simulink model "TestAttitudeControl"  (R2016b)
settings: Solver=VariableStepAuto  StartTime=0.0  StopTime=10  RelTol=1e-3
undefined symbols (not defined in the file): armed, ctrl_state, Initial, v_att_sp, v_control_mode
libraries: QuaternionLibrary x6, simulink_extras x2, simulink x1
(part 1 of 2)
settings Model: Creator=jban039  LastModifiedBy=jban039

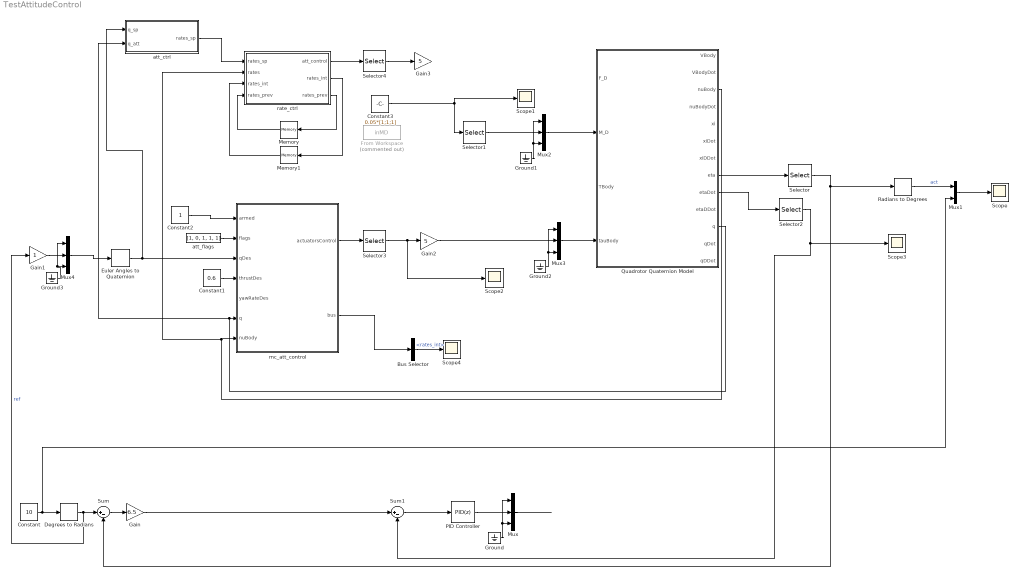
== system TestAttitudeControl ==
  Bus Selector : BusSelector  OutputSignals=rates_int
  Constant : Constant  Value=10
  Constant1 : Constant  Value=0.6
  Constant2 : Constant
  Constant3 : Constant  Value=0.05*[1;1;1]
  Degrees to Radians : simulink_extras/Transformations/Degrees to Radians
  Euler Angles to Quaternion : QuaternionLibrary/Euler Angles to Quaternion
  From Workspace : FromWorkspace  Commented=on  VariableName=inMD  SampleTime=0
  Gain : Gain  Gain=6.5
  Gain1 : Gain
  Gain2 : Gain  Gain=5
  Gain3 : Gain  Gain=5
  Ground{,1..3} (4 alike) : Ground
  Memory : Memory  X0=[0;0;0]
  Memory1 : Memory  X0=[0;0;0]
  Mux{,2..4} (4 alike) : Mux  Inputs=3
  Mux1 : Mux  Inputs=2
  PID Controller : simulink/Continuous/PID Controller  Controller=PID  TimeDomain=Discrete-time  SampleTime=0.004  IntegratorMethod=Forward Euler  FilterMethod=Forward Euler  Form=Parallel  UseFilter=off  ControllerParametersSource=internal  P=0.15  I=0.05  D=0.003  N=1000  InitialConditionSource=internal  InitialConditionForIntegrator=0  InitialConditionForFilter=0  ExternalReset=none  LimitOutput=off  UpperSaturationLimit=inf  LowerSaturationLimit=-inf  LinearizeAsGain=on  AntiWindupMode=none  Kb=1  TrackingMode=off  Kt=1  PParamMin=[]  PParamMax=[]  IParamMin=[]  IParamMax=[]  DParamMin=[]  DParamMax=[]  NParamMin=[]  NParamMax=[]  KbParamMin=[]  KbParamMax=[]  KtParamMin=[]  KtParamMax=[]  POutMin=[]  POutMax=[]  IOutMin=[]  IOutMax=[]  DOutMin=[]  DOutMax=[]  NOutMin=[]  NOutMax=[]  KbOutMin=[]  KbOutMax=[]  KtOutMin=[]  KtOutMax=[]  IntegratorOutMin=[]  IntegratorOutMax=[]  FilterOutMin=[]  FilterOutMax=[]  SumOutMin=[]  SumOutMax=[]  SumI1OutMin=[]  SumI1OutMax=[]  SumI2OutMin=[]  SumI2OutMax=[]  SumI3OutMin=[]  SumI3OutMax=[]  SumDOutMin=[]  SumDOutMax=[]  SaturationOutMin=[]  SaturationOutMax=[]  IntegratorContinuousStateAttributes=''  IntegratorStateMustResolveToSignalObject=off  IntegratorRTWStateStorageClass=Auto  FilterContinuousStateAttributes=''  FilterStateMustResolveToSignalObject=off  FilterRTWStateStorageClass=Auto  DifferentiatorICPrevScaledInput=0  DifferentiatorOutMin=[]  DifferentiatorOutMax=[]
  Quadrotor Quaternion Model : Subsystem
  Radians to Degrees : simulink_extras/Transformations/Radians to Degrees
  Scope{,1..4} (5 alike) : Scope
  Selector{,1..2,4} (4 alike) : Selector  InputPortWidth=3  IndexOptions=Index vector (dialog)  Indices=2  OutputSizes=1
  Selector3 : Selector  InputPortWidth=8  IndexOptions=Index vector (dialog)  Indices=2  OutputSizes=1
  Sum : Sum  Inputs=|+-
  Sum1 : Sum  Inputs=|+-
  att_ctrl : MATLAB Function  TreatAsAtomicUnit=on
  att_flags : Constant  Value=[1, 0, 1, 1, 1]
  mc_att_control : Subsystem  AncestorBlock=Px4Library/mc_att_control  mask(PX4 Attitude Controller: mc_att_control){MC_SAMPLING_PERIOD=0.004, MC_ROLL_TC=0.2, MC_PITCH_TC=0.2, MC_ROLL_P=6.5, MC_ROLLRATE_P=0.15, MC_ROLLRATE_I=0.05, MC_ROLLRATE_D=0.003, MC_ROLLRATE_FF=0, MC_PITCH_P=6.5, MC_PITCHRATE_P=0.15, MC_PITCHRATE_I=0.05, MC_PITCHRATE_D=0.003, MC_PITCHRATE_FF=0, MC_YAW_P=2.8, MC_YAWRATE_P=0.2, MC_YAWRATE_I=0.1, MC_YAWRATE_D=0, MC_YAWRATE_FF=0, MC_YAW_FF=0.5, MC_ROLLRATE_MAX=220, MC_PITCHRATE_MAX=220, MC_YAWRATE_MAX=200, MC_YAWRAUTO_MAX=45, MC_ACRO_R_MAX=360, MC_ACRO_P_MAX=360, MC_ACRO_Y_MAX=360, MC_RATT_TH=1, MC_TPA_BREAK=1, MC_TPA_SLOPE=1, VT_OPT_RECOV_EN=0, VT_WV_YAWR_SCL=0.15, MC_RR_INT_LIM=10.0, MC_PR_INT_LIM=10.0, MC_TPA_BREAK_P=1.0, MC_TPA_BREAK_I=1.0, MC_TPA_BREAK_D=1.0, MC_TPA_RATE_P=0.0, MC_TPA_RATE_I=0.0, MC_TPA_RATE_D=0.0, VT_TYPE=0, MC_BAT_SCALE_EN=0, MC_YR_INT_LIM=10.0}
      mask prompts: VT_TYPE "VT_TYPE (0 = Tailsitter, 1 = Tiltrotor, 2 = Standard)"
      mask help: Stabilization controller from the PX4 flight stack.
  rate_ctrl : MATLAB Function  TreatAsAtomicUnit=on  SystemSampleTime=0.002
  wires:
  Mux/1 -> ?
  Constant3/1 -> Selector1/1, Scope1/1
  Constant/1 -> Mux1/2, Degrees to Radians/1
  Sum/1 -> Gain/1
  Ground/1 -> Mux/1, Mux/3
  PID Controller/1 -> Mux/2
  Quadrotor Quaternion Model/8(eta) -> Selector/1
  Selector/1 -> Radians to Degrees/1, Sum/2
  Degrees to Radians/1 -> Gain1/1, Sum/1  "ref"
  Radians to Degrees/1 -> Mux1/1  "act"
  Mux1/1 -> Scope/1
  Ground1/1 -> Mux2/3, Mux2/1
  Selector1/1 -> Mux2/2
  Mux2/1 -> Quadrotor Quaternion Model/2(M_D)
  Quadrotor Quaternion Model/9(etaDot) -> Selector2/1
  Gain/1 -> Sum1/1
  Sum1/1 -> PID Controller/1
  mc_att_control/1(actuatorsControl) -> Selector3/1
  Euler Angles to Quaternion/1 -> att_ctrl/1(q_sp), mc_att_control/3(qDes)
  Constant1/1 -> mc_att_control/4(thrustDes)
  Quadrotor Quaternion Model/11(q) -> att_ctrl/2(q_att), mc_att_control/6(q)
  Quadrotor Quaternion Model/3(nuBody) -> rate_ctrl/2(rates), mc_att_control/7(nuBody)
  Constant2/1 -> mc_att_control/1(armed)
  att_flags/1 -> mc_att_control/2(flags)
  Mux3/1 -> Quadrotor Quaternion Model/4(tauBody)
  Ground2/1 -> Mux3/3, Mux3/1
  Selector3/1 -> Scope2/1, Gain2/1
  Mux4/1 -> Euler Angles to Quaternion/1
  Ground3/1 -> Mux4/1, Mux4/3
  Gain1/1 -> Mux4/2
  Gain2/1 -> Mux3/2
  Selector2/1 -> Scope3/1, Sum1/2
  att_ctrl/1(rates_sp) -> rate_ctrl/1(rates_sp)
  rate_ctrl/3(rates_prev) -> Memory/1
  Memory/1 -> rate_ctrl/4("rates_prev ")
  rate_ctrl/2(rates_int) -> Memory1/1
  Memory1/1 -> rate_ctrl/3("rates_int ")
  rate_ctrl/1(att_control) -> Selector4/1
  Selector4/1 -> Gain3/1
  mc_att_control/2(bus) -> Bus Selector/1
  Bus Selector/1 -> Scope4/1  "<rates_int>"

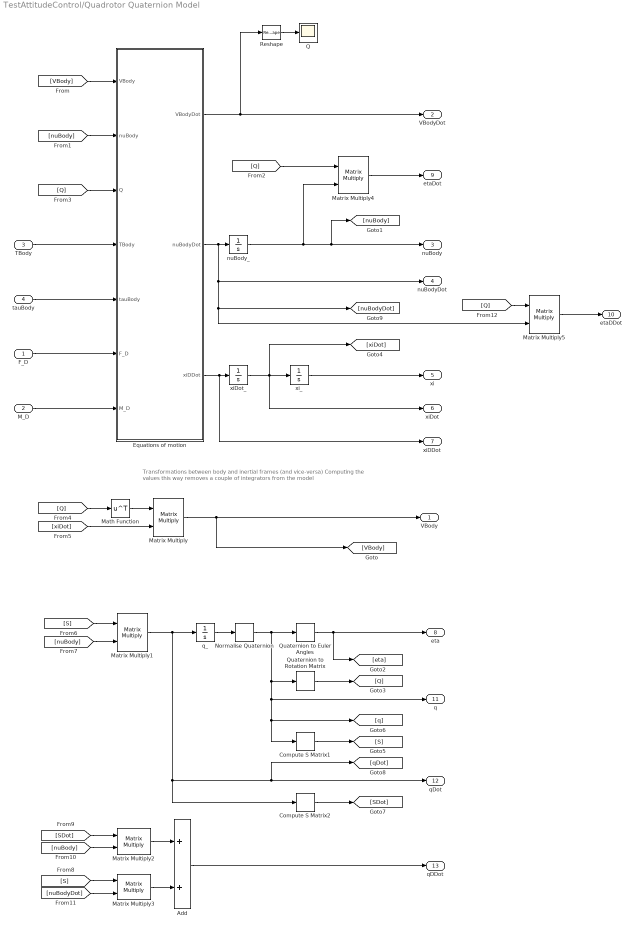
== system TestAttitudeControl/Quadrotor Quaternion Model ==
  note: Transformations between body and inertial frames (and vice-versa)
      | Computing the values this way removes a couple of integrators from the model
  F_D : Inport  Unit=N
  M_D : Inport  Port=2  Unit=N*m
  TBody : Inport  Port=3  Unit=N
  tauBody : Inport  Port=4  Unit=N*m
  Add : Sum
  Compute S Matrix1 : QuaternionLibrary/Compute S Matrix
  Compute S Matrix2 : QuaternionLibrary/Compute S Matrix
  Equations of motion : MATLAB Function  TreatAsAtomicUnit=on
  Math Function : Math  Operator=transpose  SaturateOnIntegerOverflow=on
  Matrix Multiply{,1..5} (6 alike) : Product  Multiplication=Matrix(*)
  Normalise Quaternion : QuaternionLibrary/Normalise Quaternion
  Q : Scope
  Quaternion to Euler Angles : QuaternionLibrary/Quaternion to Euler Angles
  Quaternion to Rotation Matrix : QuaternionLibrary/Quaternion to Rotation Matrix
  Reshape : Reshape  OutputDimensionality=Column vector (2-D)
  nuBody_ : Integrator  InitialCondition=Initial.NU_BODY
  q_ : Integrator  InitialCondition=Initial.Q
  xiDot_ : Integrator  InitialCondition=Initial.XI_DOT
  xi_ : Integrator  InitialCondition=Initial.XI
  VBody : Outport  Unit=m/s
  VBodyDot : Outport  Port=2  Unit=m/s^2
  nuBody : Outport  Port=3  Unit=rad/s
  nuBodyDot : Outport  Port=4  Unit=rad/s^2
  xi : Outport  Port=5  Unit=m
  xiDot : Outport  Port=6  Unit=m/s
  xiDDot : Outport  Port=7  Unit=m/s^2
  eta : Outport  Port=8  Unit=rad
  etaDot : Outport  Port=9  Unit=rad/s
  etaDDot : Outport  Port=10  Unit=rad/s^2
  q : Outport  Port=11
  qDot : Outport  Port=12
  qDDot : Outport  Port=13
  wires:
  Equations of motion/1(VBodyDot) -> Reshape/1, VBodyDot/1
  xi_/1 -> xi/1
  [nuBody] -> Equations of motion/2(nuBody)
  [VBody] -> Equations of motion/1(VBody)
  tauBody/1 -> Equations of motion/5(tauBody)
  TBody/1 -> Equations of motion/4(TBody)
  Equations of motion/3(xiDDot) -> xiDot_/1, xiDDot/1
  F_D/1 -> Equations of motion/6(F_D)
  Matrix Multiply/1 -> VBody/1, [VBody]
  M_D/1 -> Equations of motion/7(M_D)
  nuBody_/1 -> Matrix Multiply4/2, [nuBody], nuBody/1
  Equations of motion/2(nuBodyDot) -> nuBody_/1, nuBodyDot/1, Matrix Multiply5/2, [nuBodyDot]
  q_/1 -> Normalise Quaternion/1
  Quaternion to Euler Angles/1 -> eta/1, [eta]
  Matrix Multiply4/1 -> etaDot/1
  Quaternion to Rotation Matrix/1 -> [Q]
  [Q] -> Equations of motion/3(Q)
  [Q] -> Math Function/1
  [xiDot] -> Matrix Multiply/2
  Math Function/1 -> Matrix Multiply/1
  [S] -> Matrix Multiply1/1
  [nuBody] -> Matrix Multiply1/2
  Compute S Matrix2/1 -> [SDot]
  [S] -> Matrix Multiply3/1
  Matrix Multiply1/1 -> qDot/1, [qDot], Compute S Matrix2/1, q_/1
  [SDot] -> Matrix Multiply2/1
  [nuBody] -> Matrix Multiply2/2
  [nuBodyDot] -> Matrix Multiply3/2
  Matrix Multiply2/1 -> Add/1
  Matrix Multiply3/1 -> Add/2
  Normalise Quaternion/1 -> Quaternion to Euler Angles/1, q/1, Compute S Matrix1/1, [q], Quaternion to Rotation Matrix/1
  Compute S Matrix1/1 -> [S]
  [Q] -> Matrix Multiply4/1
  Add/1 -> qDDot/1
  [Q] -> Matrix Multiply5/1
  Matrix Multiply5/1 -> etaDDot/1
  Reshape/1 -> Q/1
  xiDot_/1 -> xi_/1, [xiDot], xiDot/1

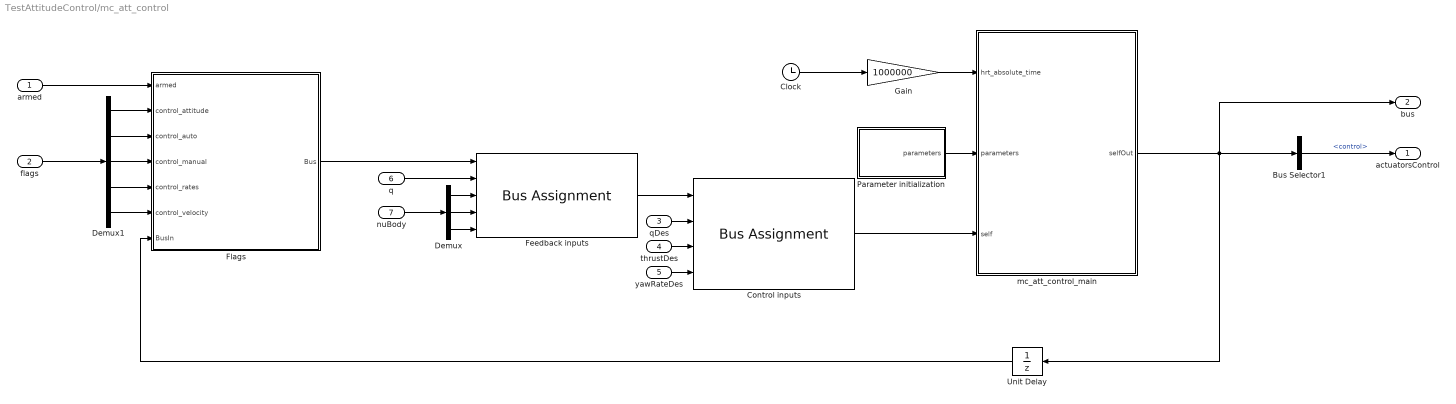
== system TestAttitudeControl/mc_att_control ==
  armed : Inport  PortDimensions=1  SampleTime=MC_SAMPLING_PERIOD
  flags : Inport  Port=2  PortDimensions=5  SampleTime=MC_SAMPLING_PERIOD
  qDes : Inport  Port=3  PortDimensions=4  SampleTime=MC_SAMPLING_PERIOD
  thrustDes : Inport  Port=4  PortDimensions=1  SampleTime=MC_SAMPLING_PERIOD
  yawRateDes : Inport  Port=5  PortDimensions=1  SampleTime=MC_SAMPLING_PERIOD
  q : Inport  Port=6  PortDimensions=4  SampleTime=MC_SAMPLING_PERIOD
  nuBody : Inport  Port=7  PortDimensions=3  SampleTime=MC_SAMPLING_PERIOD
  Bus Selector1 : BusSelector  OutputSignals=actuators.control
  Clock : Clock
  Control inputs : BusAssignment  AssignedSignals=v_att_sp.q_d,v_att_sp.thrust,v_att_sp.yaw_sp_move_rate
  Demux : Demux  Outputs=3
  Demux1 : Demux  Outputs=5
  Feedback inputs : BusAssignment  AssignedSignals=ctrl_state.q,ctrl_state.roll_rate,ctrl_state.pitch_rate,ctrl_state.yaw_rate
  Flags : Subsystem
  Gain : Gain  Gain=1000000
  Parameter initialization : Subsystem
  Unit Delay : UnitDelay  SampleTime=MC_SAMPLING_PERIOD
  mc_att_control_main : MATLAB Function  TreatAsAtomicUnit=on  SystemSampleTime=MC_SAMPLING_PERIOD
  actuatorsControl : Outport  SampleTime=MC_SAMPLING_PERIOD
  bus : Outport  Port=2  SampleTime=MC_SAMPLING_PERIOD
  wires:
  flags/1 -> Demux1/1
  nuBody/1 -> Demux/1
  q/1 -> Feedback inputs/2
  armed/1 -> Flags/1(armed)
  Demux1/1 -> Flags/2(control_attitude)
  Demux1/2 -> Flags/3(control_auto)
  Demux1/3 -> Flags/4(control_manual)
  Demux1/4 -> Flags/5(control_rates)
  Demux1/5 -> Flags/6(control_velocity)
  yawRateDes/1 -> Control inputs/4
  thrustDes/1 -> Control inputs/3
  qDes/1 -> Control inputs/2
  Feedback inputs/1 -> Control inputs/1
  Gain/1 -> mc_att_control_main/1(hrt_absolute_time)
  Clock/1 -> Gain/1
  Demux/3 -> Feedback inputs/5
  Demux/2 -> Feedback inputs/4
  Demux/1 -> Feedback inputs/3
  Flags/1(Bus) -> Feedback inputs/1
  Control inputs/1 -> mc_att_control_main/3(self)
  Unit Delay/1 -> Flags/7(BusIn)
  Bus Selector1/1 -> actuatorsControl/1  "<control>"
  Parameter initialization/1(parameters) -> mc_att_control_main/2(parameters)
  mc_att_control_main/1(selfOut) -> Bus Selector1/1, Unit Delay/1, bus/1

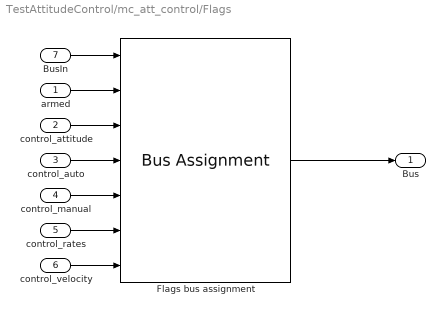
== system TestAttitudeControl/mc_att_control/Flags ==
  armed : Inport
  control_attitude : Inport  Port=2
  control_auto : Inport  Port=3
  control_manual : Inport  Port=4
  control_rates : Inport  Port=5
  control_velocity : Inport  Port=6
  BusIn : Inport  Port=7
  Flags bus assignment : BusAssignment  AssignedSignals=armed.armed,v_control_mode.flag_control_attitude_enabled,v_control_mode.flag_control_auto_enabled,v_control_mode.flag_control_manual_enabled,v_control_mode.flag_control_rates_enabled,v_control_mode.flag_control_velocity_enabled
  Bus : Outport
  wires:
  control_rates/1 -> Flags bus assignment/6
  control_manual/1 -> Flags bus assignment/5
  control_attitude/1 -> Flags bus assignment/3
  armed/1 -> Flags bus assignment/2
  control_velocity/1 -> Flags bus assignment/7
  control_auto/1 -> Flags bus assignment/4
  BusIn/1 -> Flags bus assignment/1
  Flags bus assignment/1 -> Bus/1

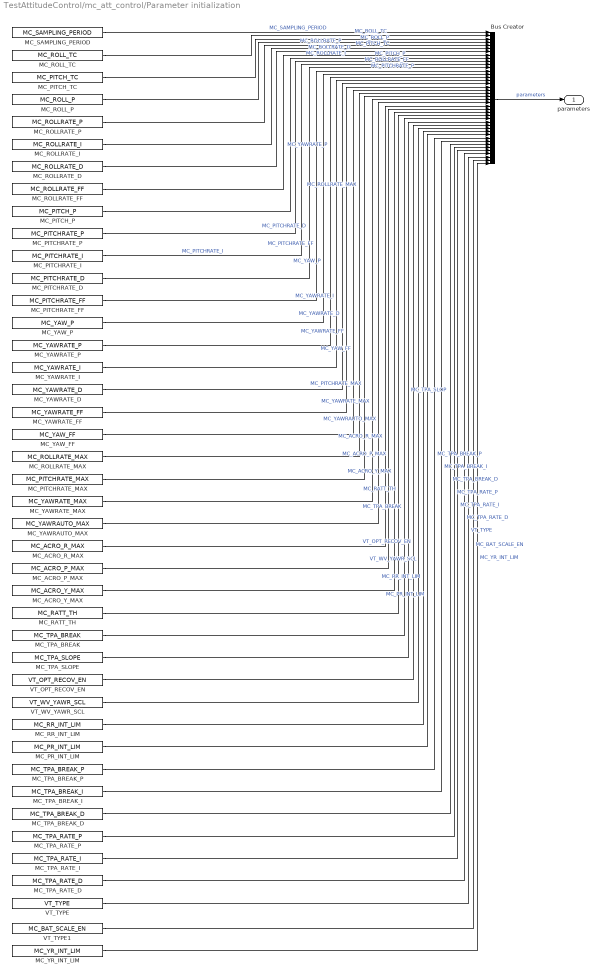
== system TestAttitudeControl/mc_att_control/Parameter initialization ==
  Bus Creator : BusCreator  Inputs='MC_SAMPLING_PERIOD','MC_ROLL_TC','MC_PITCH_TC','MC_ROLL_P','MC_ROLLRATE_P','MC_ROLLRATE_I','MC_ROLLRATE_D','MC_ROLLRATE_FF','MC_PITCH_P','MC_PITCHRATE_P','MC_PITCHRATE_I','MC_PITCHRATE_D','MC_PITCHRATE_FF','MC_YAW_P','MC_YAWRATE_P','MC_YAWRATE_I','MC_YAWRATE_D','MC_YAWRATE_FF','MC_YAW_FF','MC_ROLLRATE_MAX','MC_PITCHRATE_MAX','MC_YAWRATE_MAX','MC_YAWRAUTO_MAX','MC_ACRO_R_MAX','MC_ACRO_P_MAX','MC_ACRO_Y_MAX','MC_RATT_TH','MC_TPA_BREAK','MC_TPA_SLOP','VT_OPT_RECOV_EN','VT_WV_YAWR_SCL','MC_RR_INT_LIM','MC_PR_INT_LIM','MC_TPA_BREAK_P','MC_TPA_BREAK_I','MC_TPA_BREAK_D','MC_TPA_RATE_P','MC_TPA_RATE_I','MC_TPA_RATE_D','VT_TYPE','MC_BAT_SCALE_EN','MC_YR_INT_LIM'  OutDataTypeStr=Bus: parameterBus
  MC_ACRO_P_MAX : Constant  Value=MC_ACRO_P_MAX
  MC_ACRO_R_MAX : Constant  Value=MC_ACRO_R_MAX
  MC_ACRO_Y_MAX : Constant  Value=MC_ACRO_Y_MAX
  MC_PITCHRATE_D : Constant  Value=MC_PITCHRATE_D
  MC_PITCHRATE_FF : Constant  Value=MC_PITCHRATE_FF
  MC_PITCHRATE_I : Constant  Value=MC_PITCHRATE_I
  MC_PITCHRATE_MAX : Constant  Value=MC_PITCHRATE_MAX
  MC_PITCHRATE_P : Constant  Value=MC_PITCHRATE_P
  MC_PITCH_P : Constant  Value=MC_PITCH_P
  MC_PITCH_TC : Constant  Value=MC_PITCH_TC
  MC_PR_INT_LIM : Constant  Value=MC_PR_INT_LIM
  MC_RATT_TH : Constant  Value=MC_RATT_TH
  MC_ROLLRATE_D : Constant  Value=MC_ROLLRATE_D
  MC_ROLLRATE_FF : Constant  Value=MC_ROLLRATE_FF
  MC_ROLLRATE_I : Constant  Value=MC_ROLLRATE_I
  MC_ROLLRATE_MAX : Constant  Value=MC_ROLLRATE_MAX
  MC_ROLLRATE_P : Constant  Value=MC_ROLLRATE_P
  MC_ROLL_P : Constant  Value=MC_ROLL_P
  MC_ROLL_TC : Constant  Value=MC_ROLL_TC
  MC_RR_INT_LIM : Constant  Value=MC_RR_INT_LIM
  MC_SAMPLING_PERIOD : Constant  Value=MC_SAMPLING_PERIOD
  MC_TPA_BREAK : Constant  Value=MC_TPA_BREAK
  MC_TPA_BREAK_D : Constant  Value=MC_TPA_BREAK_D
  MC_TPA_BREAK_I : Constant  Value=MC_TPA_BREAK_I
  MC_TPA_BREAK_P : Constant  Value=MC_TPA_BREAK_P
  MC_TPA_RATE_D : Constant  Value=MC_TPA_RATE_D
  MC_TPA_RATE_I : Constant  Value=MC_TPA_RATE_I
  MC_TPA_RATE_P : Constant  Value=MC_TPA_RATE_P
  MC_TPA_SLOPE : Constant  Value=MC_TPA_SLOPE
  MC_YAWRATE_D : Constant  Value=MC_YAWRATE_D
  MC_YAWRATE_FF : Constant  Value=MC_YAWRATE_FF
  MC_YAWRATE_I : Constant  Value=MC_YAWRATE_I
  MC_YAWRATE_MAX : Constant  Value=MC_YAWRATE_MAX
  MC_YAWRATE_P : Constant  Value=MC_YAWRATE_P
  MC_YAWRAUTO_MAX : Constant  Value=MC_YAWRAUTO_MAX
  MC_YAW_FF : Constant  Value=MC_YAW_FF
  MC_YAW_P : Constant  Value=MC_YAW_P
  MC_YR_INT_LIM : Constant  Value=MC_YR_INT_LIM
  VT_OPT_RECOV_EN : Constant  Value=VT_OPT_RECOV_EN
  VT_TYPE : Constant  Value=VT_TYPE
  VT_TYPE1 : Constant  Value=MC_BAT_SCALE_EN
  VT_WV_YAWR_SCL : Constant  Value=VT_WV_YAWR_SCL
  parameters : Outport
  wires:
  MC_RR_INT_LIM/1 -> Bus Creator/32  "MC_RR_INT_LIM"
  VT_TYPE1/1 -> Bus Creator/41  "MC_BAT_SCALE_EN"
  MC_TPA_BREAK_D/1 -> Bus Creator/36  "MC_TPA_BREAK_D"
  MC_TPA_BREAK_I/1 -> Bus Creator/35  "MC_TPA_BREAK_I"
  MC_TPA_BREAK_P/1 -> Bus Creator/34  "MC_TPA_BREAK_P"
  MC_YR_INT_LIM/1 -> Bus Creator/42  "MC_YR_INT_LIM"
  MC_TPA_RATE_D/1 -> Bus Creator/39  "MC_TPA_RATE_D"
  VT_TYPE/1 -> Bus Creator/40  "VT_TYPE"
  MC_TPA_BREAK/1 -> Bus Creator/28  "MC_TPA_BREAK"
  VT_WV_YAWR_SCL/1 -> Bus Creator/31  "VT_WV_YAWR_SCL"
  MC_TPA_SLOPE/1 -> Bus Creator/29  "MC_TPA_SLOP"
  MC_ACRO_R_MAX/1 -> Bus Creator/24  "MC_ACRO_R_MAX"
  Bus Creator/1 -> parameters/1  "parameters"
  MC_ACRO_P_MAX/1 -> Bus Creator/25  "MC_ACRO_P_MAX"
  MC_ACRO_Y_MAX/1 -> Bus Creator/26  "MC_ACRO_Y_MAX"
  VT_OPT_RECOV_EN/1 -> Bus Creator/30  "VT_OPT_RECOV_EN"
  MC_RATT_TH/1 -> Bus Creator/27  "MC_RATT_TH"
  MC_YAWRATE_MAX/1 -> Bus Creator/22  "MC_YAWRATE_MAX"
  MC_YAWRAUTO_MAX/1 -> Bus Creator/23  "MC_YAWRAUTO_MAX"
  MC_YAWRATE_P/1 -> Bus Creator/15  "MC_YAWRATE_P"
  MC_ROLL_TC/1 -> Bus Creator/2  "MC_ROLL_TC"
  MC_PITCH_P/1 -> Bus Creator/9  "MC_PITCH_P"
  MC_PITCH_TC/1 -> Bus Creator/3  "MC_PITCH_TC"
  MC_SAMPLING_PERIOD/1 -> Bus Creator/1  "MC_SAMPLING_PERIOD"
  MC_PITCHRATE_MAX/1 -> Bus Creator/21  "MC_PITCHRATE_MAX"
  MC_YAWRATE_I/1 -> Bus Creator/16  "MC_YAWRATE_I"
  MC_ROLL_P/1 -> Bus Creator/4  "MC_ROLL_P"
  MC_ROLLRATE_MAX/1 -> Bus Creator/20  "MC_ROLLRATE_MAX"
  MC_YAW_P/1 -> Bus Creator/14  "MC_YAW_P"
  MC_YAWRATE_FF/1 -> Bus Creator/18  "MC_YAWRATE_FF"
  MC_ROLLRATE_FF/1 -> Bus Creator/8  "MC_ROLLRATE_FF"
  MC_PITCHRATE_D/1 -> Bus Creator/12  "MC_PITCHRATE_D"
  MC_PITCHRATE_I/1 -> Bus Creator/11  "MC_PITCHRATE_I"
  MC_ROLLRATE_D/1 -> Bus Creator/7  "MC_ROLLRATE_D"
  MC_ROLLRATE_P/1 -> Bus Creator/5  "MC_ROLLRATE_P"
  MC_PITCHRATE_P/1 -> Bus Creator/10  "MC_PITCHRATE_P"
  MC_PITCHRATE_FF/1 -> Bus Creator/13  "MC_PITCHRATE_FF"
  MC_YAW_FF/1 -> Bus Creator/19  "MC_YAW_FF"
  MC_YAWRATE_D/1 -> Bus Creator/17  "MC_YAWRATE_D"
  MC_ROLLRATE_I/1 -> Bus Creator/6  "MC_ROLLRATE_I"
  MC_PR_INT_LIM/1 -> Bus Creator/33  "MC_PR_INT_LIM"
  MC_TPA_RATE_P/1 -> Bus Creator/37  "MC_TPA_RATE_P"
  MC_TPA_RATE_I/1 -> Bus Creator/38  "MC_TPA_RATE_I"

== matlab function TestAttitudeControl/Quadrotor Quaternion Model/Equations of motion ==
  data: VBody input; VBodyDot output; nuBody input; Q input; TBody input size=3; tauBody input size=3; F_D input size=3; M_D input size=3; nuBodyDot output; Uav parameter; xiDDot output
function [VBodyDot, nuBodyDot, xiDDot] = QuadrotorQuaternionModel(...
    VBody, nuBody, Q, TBody, tauBody, F_D, M_D, Uav)
%#codegen

%% Rotation matrices

%% Moments and Forces
% Body frame accelerations
VBodyDot  = (1/Uav.M) * (Q'*Uav.G + TBody - cross(nuBody, Uav.M*VBody) - F_D);
nuBodyDot = Uav.I \ (tauBody - cross(nuBody, Uav.I*nuBody) - M_D);

% Inertial frame accelerations
xiDDot = (1/Uav.M)*(Uav.G + Q*(TBody - F_D));
% etaDDot = WInvertDot*nuBody + WInvert*nuBodyDot;

% Check centripetal force in inertial frame
% F_C = R*cross(nuBody,m*VBody);
end

== matlab function TestAttitudeControl/att_ctrl ==
  data: q_sp input size=4; rates_sp output size=3; q_att input size=4
function rates_sp = att_ctrl(q_sp, q_att)
%#codegen

    R_sp  = QuatToRot( q_sp );
    R     = QuatToRot( q_att );
    att_p = [6.5; 6.5; 2.8];

    % Try to move thrust vector shortest way, because yaw response is slower than roll/pitch
    R_z = R(:,3);
    R_sp_z = R_sp(:,3);
    
    % Axis and sin(angle) of desired rotation
    e_R = R' * cross(R_z, R_sp_z);             % sin theta * n

    % Calculate angle error
    e_R_z_sin = norm(e_R);                     % sin theta
    e_R_z_cos = dot(R_z, R_sp_z);              % cos theta

    % Calculate rotation matrix after roll/pitch only rotation
    if ( e_R_z_sin > 0.0 )
        e_R_z_angle = atan2(e_R_z_sin, e_R_z_cos); % theta
        e_R_z_axis = e_R ./ e_R_z_sin;             % n

        e_R = e_R_z_axis .* e_R_z_angle;           % e_R
        % Cross product matrix for e_R_axis
        e_R_cp = zeros(3,3); % E_R
        e_R_cp(1, 2) = -e_R_z_axis(3);
        e_R_cp(1, 3) =  e_R_z_axis(2);
        e_R_cp(2, 1) =  e_R_z_axis(3);
        e_R_cp(2, 3) = -e_R_z_axis(1);
        e_R_cp(3, 1) = -e_R_z_axis(2);
        e_R_cp(3, 2) =  e_R_z_axis(1);

        % Rotation matrix for roll/pitch only rotation
        R_rp = R * ( eye(3,3) + e_R_cp * e_R_z_sin + e_R_cp * e_R_cp * (1.0 - e_R_z_cos) );
    else
        % Zero roll/pitch rotation
        R_rp = R;
    end

    % Calculate weight for yaw control
    yaw_w = R_sp(3, 3) * R_sp(3, 3); % w_psi

    % R_rp and R_sp has the same Z axis, calculate yaw error
    R_sp_x = R_sp(:, 1);
    R_rp_x = R_rp(:, 1);
    e_R(3) = atan2( dot( cross(R_rp_x, R_sp_x), R_sp_z), dot(R_rp_x, R_sp_x) ) * yaw_w;

    if ( e_R_z_cos < 0.0 )
        % For large thrust vector rotations use another rotation method:
        % calculate angle and axis for R -> R_sp rotation directly
        q_error = RotToQuat( R' * R_sp );

        if ( q_error(1) >= 0.0 )
            e_R_d =  q_error(2:end) * 2.0; % Still not 100% sure
        else
            e_R_d = -q_error(2:end) * 2.0;
        end


        % Use fusion of Z axis based rotation and direct rotation
        direct_w = e_R_z_cos * e_R_z_cos * yaw_w;
        e_R = e_R * (1.0 - direct_w) + e_R_d * direct_w;
    end

    rates_sp = att_p .* e_R;
    
end

function R = QuatToRot( q )
% QUATERNIONTOROTATIONMATRIXMAT Convert quaternion to rotation matrix
% Written by: J.X.J. Bannwarth, 27/03/17
    W = q(1);
    X = q(2);
    Y = q(3);
    Z = q(4);
    
    xx = X * X;
    xy = X * Y;
    xz = X * Z;
    xw = X * W;

    yy = Y * Y;
    yz = Y * Z;
    yw = Y * W;
    
    zz = Z * Z;
    zw = Z * W;

    m00 = 1 - 2 * ( yy + zz );
    m01 =     2 * ( xy - zw );
    m02 =     2 * ( xz + yw );

    m10 =     2 * ( xy + zw );
    m11 = 1 - 2 * ( xx + zz );
    m12 =     2 * ( yz - xw );

    m20 =     2 * ( xz - yw );
    m21 =     2 * ( yz + xw );
    m22 = 1 - 2 * ( xx + yy );
    
    R = [m00 m01 m02;
         m10 m11 m12;
         m20 m21 m22];
    
end

== matlab function TestAttitudeControl/rate_ctrl ==
  data: rates_sp input size=3; rates input size=[3,1]; att_control output size=3; rates_int output; rates_prev output; rates_int input size=3; rates_prev input size=3
function [ att_control, rates_int, rates_prev ] = rate_ctrl(rates_sp, rates, rates_int, rates_prev)
rates_p = [0.15; 0.15; 0.2];
rates_i = [0.05; 0.05; 0.1];
rates_d = [0.003; 0.003; 0];
rate_ff = [0; 0; 0];
dt = 0.002;
% Angular rates error
rates_err = rates_sp - rates;

% Perform the integration using a first order method and do not propaate the result if out of range or invalid
rates_int = rates_int + rates_i .* rates_err * dt;

att_control = rates_p .* rates_err + rates_int + rates_d .* (rates_prev - rates) ./ dt + rate_ff .* rates_sp;

rates_prev = rates;

end
